simulink model "quadricopter"  (Simulink 8.1)
settings: Solver=ode3  StartTime=0.0  StopTime=10  FixedStep=0.0005  RelTol=1e-5
values from neighbouring files (symbols this model uses):
  u1 = 0.0001    [quad_init.m]
  u2 = 0.00008    (= 8e-05)    [quad_init.m]
  u3 = 0.00009    (= 9e-05)    [quad_init.m]
  u4 = 0.00009    (= 9e-05)    [quad_init.m]
libraries: quad_lib x1
settings Model: Creator=diogo  LastModifiedBy=diogo
settings DataIOCC: LimitDataPoints=off
settings DebuggingCC: StrictBusMsg=Warning

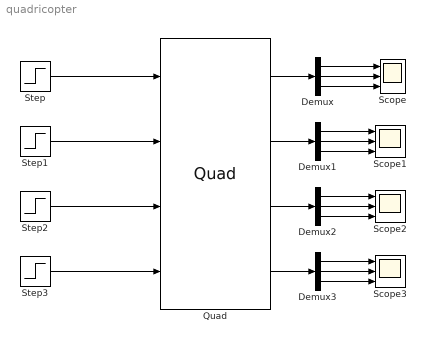
== system quadricopter ==
  Demux{,1..3} (4 alike) : Demux  Outputs=3
  Quad : quad_lib/Quad
  Scope{,1..3} (4 alike) : Scope  NumInputPorts=3
      Scope settings: YMin=-5~-5~-5  YMax=5~5~5
      Scope1 settings: YMin=-5~-5~-5  YMax=5~5~5
      Scope2 settings: YMin=-5~-5~-5  YMax=5~5~5  SaveName=ScopeData2
      Scope3 settings: YMin=-5~-5~-5  YMax=5~5~5  SaveName=ScopeData3
  Step : Step  Time=0  After=u1  SampleTime=0
  Step1 : Step  Time=0  After=u2  SampleTime=0
  Step2 : Step  Time=0  After=u3  SampleTime=0
  Step3 : Step  Time=0  After=u4  SampleTime=0
  wires:
  Step/1 -> Quad/1
  Step1/1 -> Quad/2
  Step2/1 -> Quad/3
  Step3/1 -> Quad/4
  Demux/1 -> Scope/1
  Demux/2 -> Scope/2
  Demux/3 -> Scope/3
  Quad/1 -> Demux/1
  Quad/2 -> Demux1/1
  Demux1/1 -> Scope1/1
  Demux1/2 -> Scope1/2
  Demux1/3 -> Scope1/3
  Quad/3 -> Demux2/1
  Demux2/1 -> Scope2/1
  Demux2/2 -> Scope2/2
  Demux2/3 -> Scope2/3
  Demux3/1 -> Scope3/1
  Demux3/2 -> Scope3/2
  Demux3/3 -> Scope3/3
  Quad/4 -> Demux3/1
